simulink model "CEngDsT_VD"  (R2018a)
settings: configuration reference "cs_ert" (kept outside this file)
model workspace (MAT data in the model file):
  CEngDsT_VD_DT = 10
values from neighbouring files (symbols this model uses):
  CEngDsT_facSerPT1_C = 50.0    [CEngDsT_VD.sldd]
  CEngDsT_RmpSlpNeg_C = 3.0    [CEngDsT_VD.sldd]
  CEngDsT_RmpSlpPos_C = 3.0    [CEngDsT_VD.sldd]
  CEngDsT_tDflCold_C = 10.0    [CEngDsT_VD.sldd]
  CEngDsT_tDflWarm_C = 100.0    [CEngDsT_VD.sldd]
  SigTst_swtCEngDsT_C = 0    [CEngDsT_VD.sldd]
  SigTst_tCEngDsT_C = 20.0    [CEngDsT_VD.sldd]
undefined symbols (not defined in the file or in its folder): EngState, Switch
libraries: sllib x2
settings Model: DataDictionary=CEngDsT_VD.sldd  Creator=zhoutinglin  LastModifiedBy=zhoutinglin

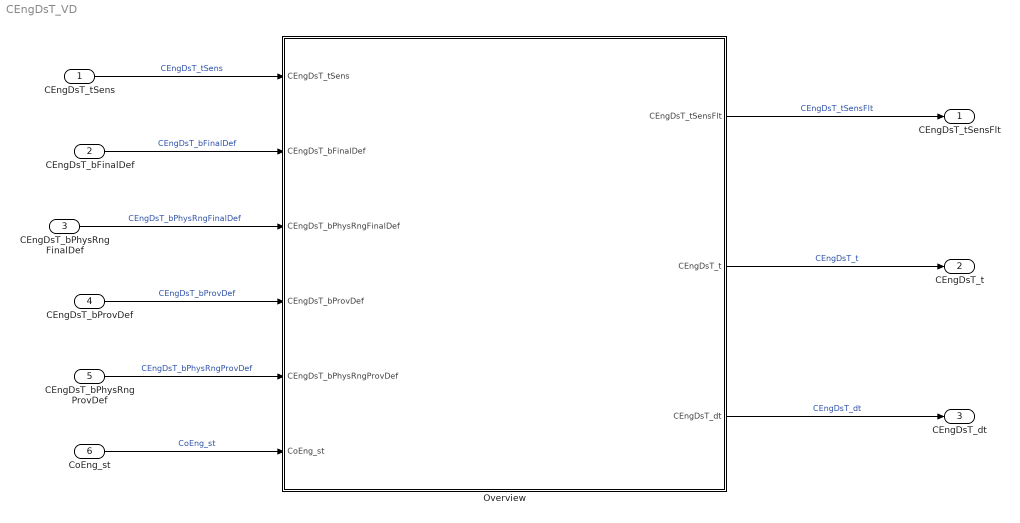
== system CEngDsT_VD ==
  CEngDsT_tSens : Inport  Tag=[]  Description=[]
  CEngDsT_bFinalDef : Inport  Tag=[]  Description=[]  Port=2
  CEngDsT_bPhysRngFinalDef : Inport  Tag=[]  Description=[]  Port=3
  CEngDsT_bProvDef : Inport  Tag=[]  Description=[]  Port=4
  CEngDsT_bPhysRngProvDef : Inport  Tag=[]  Description=[]  Port=5
  CoEng_st : Inport  Tag=[]  Description=[]  Port=6
  Overview : Subsystem
  CEngDsT_tSensFlt : Outport  Tag=[]  Description=[]
  CEngDsT_t : Outport  Tag=[]  Description=[]  Port=2
  CEngDsT_dt : Outport  Tag=[]  Description=[]  Port=3
  wires:
  Overview/3(CEngDsT_dt) -> CEngDsT_dt/1  "CEngDsT_dt"
  Overview/1(CEngDsT_tSensFlt) -> CEngDsT_tSensFlt/1  "CEngDsT_tSensFlt"
  CEngDsT_bPhysRngProvDef/1 -> Overview/5(CEngDsT_bPhysRngProvDef)  "CEngDsT_bPhysRngProvDef"
  CEngDsT_bFinalDef/1 -> Overview/2(CEngDsT_bFinalDef)  "CEngDsT_bFinalDef"
  CEngDsT_bPhysRngFinalDef/1 -> Overview/3(CEngDsT_bPhysRngFinalDef)  "CEngDsT_bPhysRngFinalDef"
  CoEng_st/1 -> Overview/6(CoEng_st)  "CoEng_st"
  CEngDsT_bProvDef/1 -> Overview/4(CEngDsT_bProvDef)  "CEngDsT_bProvDef"
  CEngDsT_tSens/1 -> Overview/1(CEngDsT_tSens)  "CEngDsT_tSens"
  Overview/2(CEngDsT_t) -> CEngDsT_t/1  "CEngDsT_t"

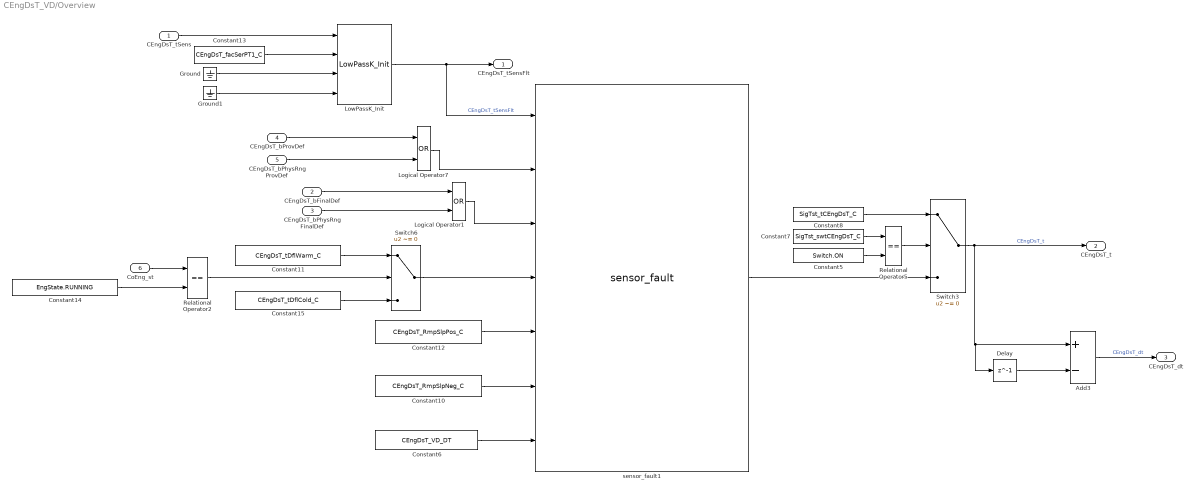
== system CEngDsT_VD/Overview ==
  CEngDsT_tSens : Inport  Tag=deg  Description=Sensed engine coolant temperature  OutMin=-200  OutMax=200
  CEngDsT_bFinalDef : Inport  Description=Status Sensor of the coolant temperature finally defect  Port=2  OutMin=0  OutMax=1  OutDataTypeStr=boolean
  CEngDsT_bPhysRngFinalDef : Inport  Description=Status Sensor of the CEngDsT physical Signal range check finally defect  Port=3  OutMin=0  OutMax=1  OutDataTypeStr=boolean
  CEngDsT_bProvDef : Inport  Description=Status Sensor of the coolant temperature temporary defect  Port=4  OutMin=0  OutMax=1  OutDataTypeStr=boolean
  CEngDsT_bPhysRngProvDef : Inport  Description=Status Sensor of the CEngDsT physical Signal range check temporary defect  Port=5  OutMin=0  OutMax=1  OutDataTypeStr=boolean
  CoEng_st : Inport  Description=Engine coordinator state  Port=6
  Add3 : Sum  Inputs=+-  OutDataTypeStr=Inherit: Inherit via back propagation  InputSameDT=on
  Constant10 : Constant  Value=CEngDsT_RmpSlpNeg_C  SampleTime=-1
  Constant11 : Constant  Value=CEngDsT_tDflWarm_C  SampleTime=-1
  Constant12 : Constant  Value=CEngDsT_RmpSlpPos_C  SampleTime=-1
  Constant13 : Constant  Value=CEngDsT_facSerPT1_C  SampleTime=-1
  Constant14 : Constant  Value=EngState.RUNNING  OutDataTypeStr=Enum: EngState
  Constant15 : Constant  Value=CEngDsT_tDflCold_C  SampleTime=-1
  Constant5 : Constant  Value=Switch.ON  OutDataTypeStr=Enum: Switch
  Constant6 : Constant  Value=CEngDsT_VD_DT  SampleTime=-1
  Constant7 : Constant  Value=SigTst_swtCEngDsT_C  SampleTime=-1
  Constant8 : Constant  Value=SigTst_tCEngDsT_C  SampleTime=-1
  Delay : Delay  DialogController=Simulink.DDGSource  DelayLength=1  InitialCondition=0
  Ground : Ground
  Ground1 : Ground
  Logical Operator1 : Logic  Operator=OR  OutDataTypeStr=boolean
  Logical Operator7 : Logic  Operator=OR  OutDataTypeStr=boolean
  LowPassK_Init : sllib/LowPassK_Init
      settings: SourceProductName=sllib
  Relational Operator2 : RelationalOperator  Operator===  OutDataTypeStr=boolean  RndMeth=Nearest  InputSameDT=on
  Relational Operator5 : RelationalOperator  Operator===  OutDataTypeStr=boolean  RndMeth=Simplest  InputSameDT=on
  Switch3 : Switch  Criteria=u2 ~= 0  InputSameDT=on
  Switch6 : Switch  Criteria=u2 ~= 0  InputSameDT=on
  sensor_fault1 : sllib/sensor_fault
      settings: SourceProductName=sllib
  CEngDsT_tSensFlt : Outport  Tag=deg  Description=engine coolant sensor temperature without speed up  OutMin=-200  OutMax=200
  CEngDsT_t : Outport  Tag=deg  Description=engine coolant temperature after filter  Port=2  OutMin=-200  OutMax=200
  CEngDsT_dt : Outport  Tag=deg/s  Description=temperature change rate  Port=3  OutMin=-200  OutMax=200
  wires:
  CEngDsT_tSens/1 -> LowPassK_Init/1
  Delay/1 -> Add3/2
  Constant11/1 -> Switch6/1
  Relational Operator2/1 -> Switch6/2
  Logical Operator1/1 -> sensor_fault1/3
  Constant10/1 -> sensor_fault1/6
  Switch3/1 -> CEngDsT_t/1, Delay/1, Add3/1  "CEngDsT_t"
  Constant8/1 -> Switch3/1
  Add3/1 -> CEngDsT_dt/1  "CEngDsT_dt"
  CEngDsT_bFinalDef/1 -> Logical Operator1/1
  Ground1/1 -> LowPassK_Init/4
  Constant15/1 -> Switch6/3
  Logical Operator7/1 -> sensor_fault1/2
  Ground/1 -> LowPassK_Init/3
  Constant14/1 -> Relational Operator2/2
  Constant7/1 -> Relational Operator5/1
  Relational Operator5/1 -> Switch3/2
  Constant12/1 -> sensor_fault1/5
  LowPassK_Init/1 -> sensor_fault1/1, CEngDsT_tSensFlt/1  "CEngDsT_tSensFlt"
  sensor_fault1/1 -> Switch3/3
  CEngDsT_bProvDef/1 -> Logical Operator7/1
  CEngDsT_bPhysRngProvDef/1 -> Logical Operator7/2
  CEngDsT_bPhysRngFinalDef/1 -> Logical Operator1/2
  Constant6/1 -> sensor_fault1/7
  Switch6/1 -> sensor_fault1/4
  CoEng_st/1 -> Relational Operator2/1
  Constant5/1 -> Relational Operator5/2
  Constant13/1 -> LowPassK_Init/2
